simulink model "EE_Var_Nat_x_FCC"  (R2022b)
settings: Solver=ode45  StartTime=0.0  StopTime=5  RelTol=1e-8  EnableMultiTasking=on
settings Model: Creator=Adolfo  LastModifiedBy=adolfo
settings SolverCC: AlgebraicLoopSolver=TrustRegion
settings DataIOCC: LimitDataPoints=on  SaveFormat=Array  SignalLoggingSaveFormat=ModelDataLogs  ReturnWorkspaceOutputs=off
settings OptimizationCC: ExpressionDepthLimit=2147483647  LifeSpan=inf
settings DebuggingCC: UnderspecifiedInitializationDetection=Classic  MergeDetectMultiDrivingBlocksExec=none  SolverPrmCheckMsg=warning  FcnCallInpInsideContextMsg=warning  UnconnectedInputMsg=warning  UnconnectedOutputMsg=warning  UnconnectedLineMsg=warning  StateNameClashWarn=warning  SFUnexpectedBacktrackingDiag=warning  SFNoUnconditionalDefaultTransitionDiag=warning  SFExecutionAtInitializationDiag=none  SFMachineParentedDataDiag=warning  ArithmeticOperatorsInVariantConditions=warning
settings HardwareCC: ProdBitPerPointer=32  ProdBitPerSizeT=32  ProdBitPerPtrDiffT=32  ProdLargestAtomicFloat=None  ProdIntDivRoundTo=Undefined  ProdEndianess=Unspecified  ProdWordSize=32  ProdHWDeviceType=32-bit Generic
settings ModelReferenceCC: PropagateSignalLabelsOutOfModel=off
settings SFSimCC: SimUseLocalCustomCode=off  CustomCodeUndefinedFunction=UseInterfaceOnly
settings RTWCC: RTWUseLocalCustomCode=off
settings CodeAppCC: StateflowObjectComments=on
settings GRTTargetCC: TargetLangStandard=C89/C90 (ANSI)  CombineOutputUpdateFcns=off  GRTInterface=on
settings ConfigComp: CovMetricSettings=dw  CovSaveCumulativeToWorkspaceVar=on  CovSaveSingleToWorkspaceVar=on  CovExternalEMLEnable=off

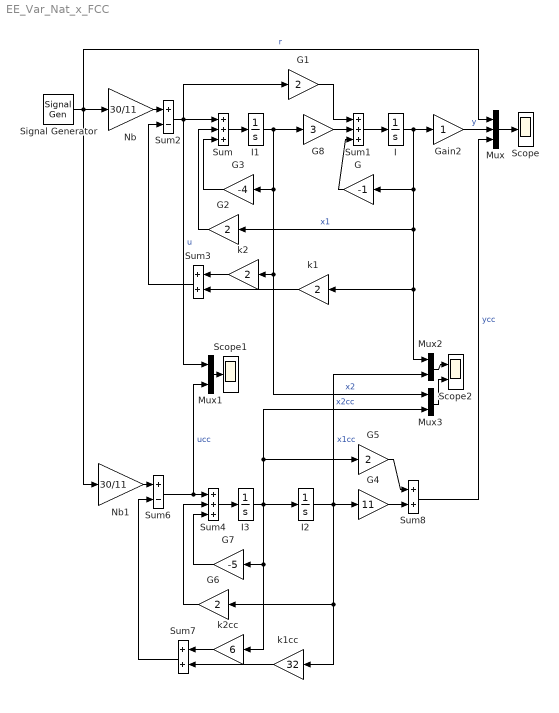
== system EE_Var_Nat_x_FCC ==
  G : Gain  Gain=-1
  G{1..2,5..6} (4 alike) : Gain  Gain=2
  G3 : Gain  Gain=-4
  G4 : Gain  Gain=11
  G7 : Gain  Gain=-5
  G8 : Gain  Gain=3
  Gain2 : Gain
  I{,1..3} (4 alike) : Integrator
  Mux : Mux  Inputs=3
  Mux1 : Mux  Inputs=2
  Mux2 : Mux  Inputs=2
  Mux3 : Mux  Inputs=2
  Nb : Gain  Gain=30/11
  Nb1 : Gain  Gain=30/11
  Scope : Scope
  Scope1 : Scope
  Scope2 : Scope  NumInputPorts=2
  Signal Generator : SignalGenerator  WaveForm=square  Frequency=.2
  Sum : Sum  Inputs=+++
  Sum1 : Sum  Inputs=+++
  Sum2 : Sum  Inputs=+-
  Sum3 : Sum
  Sum4 : Sum  Inputs=+++
  Sum6 : Sum  Inputs=+-
  Sum7 : Sum
  Sum8 : Sum
  k1 : Gain  Gain=2
  k1cc : Gain  Gain=32
  k2 : Gain  Gain=2
  k2cc : Gain  Gain=6
  wires:
  Signal Generator/1 -> Nb/1, Nb1/1, Mux/1  "r"
  Mux/1 -> Scope/1
  I/1 -> G/1, G2/1, k1/1, Mux2/1, Gain2/1  "x1"
  Sum8/1 -> Mux/3  "ycc"
  Mux1/1 -> Scope1/1
  I1/1 -> G8/1, G3/1, k2/1, Mux3/1  "x2"
  Sum/1 -> I1/1
  Sum1/1 -> I/1
  Nb/1 -> Sum2/1
  Sum2/1 -> Sum/1, G1/1, Mux1/1  "u"
  G1/1 -> Sum1/1
  G8/1 -> Sum1/2
  G/1 -> Sum1/3
  G2/1 -> Sum/2
  G3/1 -> Sum/3
  k2/1 -> Sum3/1
  k1/1 -> Sum3/2
  Sum3/1 -> Sum2/2
  I2/1 -> G4/1, G6/1, k1cc/1, Mux2/2  "x1cc"
  I3/1 -> G7/1, k2cc/1, I2/1, G5/1, Mux3/2  "x2cc"
  Sum4/1 -> I3/1
  Nb1/1 -> Sum6/1
  Sum6/1 -> Sum4/1, Mux1/2  "ucc"
  G6/1 -> Sum4/2
  G7/1 -> Sum4/3
  k2cc/1 -> Sum7/1
  k1cc/1 -> Sum7/2
  Sum7/1 -> Sum6/2
  G5/1 -> Sum8/1
  G4/1 -> Sum8/2
  Gain2/1 -> Mux/2  "y"
  Mux2/1 -> Scope2/1
  Mux3/1 -> Scope2/2
